simulink model "Series_connected_PV_modules"  (Simulink 8.4)
settings: Solver=FixedStepDiscrete  StartTime=0.0  StopTime=1  FixedStep=1e-4  RelTol=1e-3
libraries: simulink x1
(part 1 of 2)
settings Model: Creator=amaki  LastModifiedBy=lappalak
settings DebuggingCC: AlgebraicLoopMsg=none  StrictBusMsg=Warning
settings ConfigurationSet: Description=SimMechanics 2G

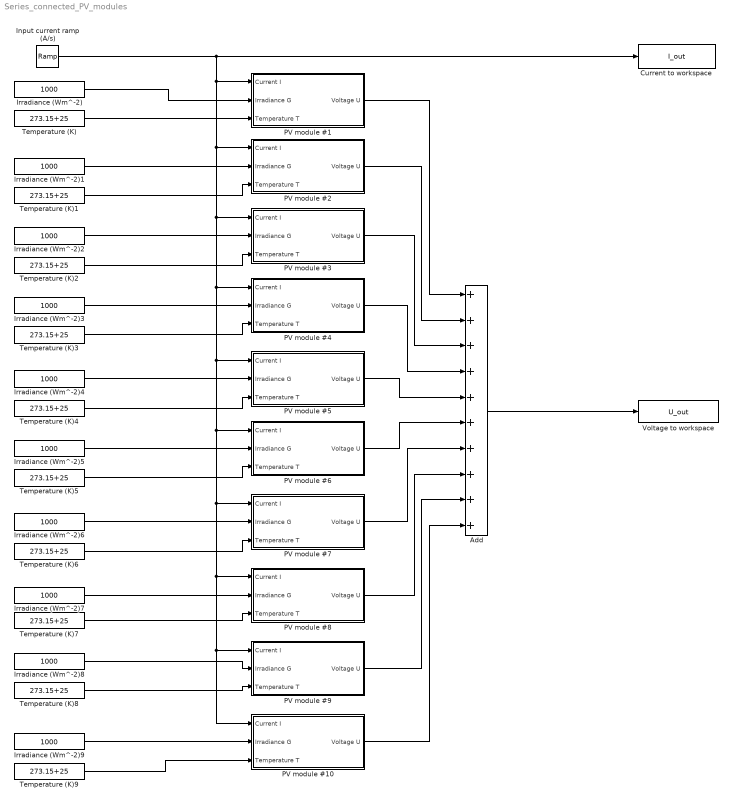
== system Series_connected_PV_modules ==
  Add : Sum  Inputs=++++++++++
  Current to workspace : ToWorkspace  VariableName=I_out  SampleTime=-1
  Input current ramp (A/s) : simulink/Sources/Ramp  slope=10  start=0  X0=0
  Irradiance (Wm^-2){,1..9} (10 alike) : Constant  Value=1000
  PV module #1 : Subsystem  mask{Isc_stc=8.02, Uoc_stc=33.1, G_stc=1000, T_stc=273.15+25, Ns=54, Rs=0.33, Rsh=188, A=1.3, Ku=-0.1242, Ki=0.0047, k=1.3806503e-23, q=1.60217646e-19}
      mask prompts: Isc_stc "STC short-circuit current"; Uoc_stc "STC open-circuit voltage"; G_stc "STC irradiance"; T_stc "STC temperature"; Ns "Number of cells"; Rs "Series resistance Rs"; Rsh "Shunt resistance Rsh"; A "Ideality factor A"; Ku "Temp. coeff. of OC Ku"; Ki "Temp. coeff. of SC Ki"; k "Boltzmann constant"; q "Elementary charge"
  PV module #10 : Subsystem  mask{Isc_stc=8.02, Uoc_stc=33.1, G_stc=1000, T_stc=273.15+25, Ns=54, Rs=0.33, Rsh=188, A=1.3, Ku=-0.1242, Ki=0.0047, k=1.3806503e-23, q=1.60217646e-19}
      mask prompts: Isc_stc "STC short-circuit current"; Uoc_stc "STC open-circuit voltage"; G_stc "STC irradiance"; T_stc "STC temperature"; Ns "Number of cells"; Rs "Series resistance Rs"; Rsh "Shunt resistance Rsh"; A "Ideality factor A"; Ku "Temp. coeff. of OC Ku"; Ki "Temp. coeff. of SC Ki"; k "Boltzmann constant"; q "Elementary charge"
  PV module #2 : Subsystem  mask{Isc_stc=8.02, Uoc_stc=33.1, G_stc=1000, T_stc=273.15+25, Ns=54, Rs=0.33, Rsh=188, A=1.3, Ku=-0.1242, Ki=0.0047, k=1.3806503e-23, q=1.60217646e-19}
      mask prompts: Isc_stc "STC short-circuit current"; Uoc_stc "STC open-circuit voltage"; G_stc "STC irradiance"; T_stc "STC temperature"; Ns "Number of cells"; Rs "Series resistance Rs"; Rsh "Shunt resistance Rsh"; A "Ideality factor A"; Ku "Temp. coeff. of OC Ku"; Ki "Temp. coeff. of SC Ki"; k "Boltzmann constant"; q "Elementary charge"
  PV module #3 : Subsystem  mask{Isc_stc=8.02, Uoc_stc=33.1, G_stc=1000, T_stc=273.15+25, Ns=54, Rs=0.33, Rsh=188, A=1.3, Ku=-0.1242, Ki=0.0047, k=1.3806503e-23, q=1.60217646e-19}
      mask prompts: Isc_stc "STC short-circuit current"; Uoc_stc "STC open-circuit voltage"; G_stc "STC irradiance"; T_stc "STC temperature"; Ns "Number of cells"; Rs "Series resistance Rs"; Rsh "Shunt resistance Rsh"; A "Ideality factor A"; Ku "Temp. coeff. of OC Ku"; Ki "Temp. coeff. of SC Ki"; k "Boltzmann constant"; q "Elementary charge"
  PV module #4 : Subsystem  mask{Isc_stc=8.02, Uoc_stc=33.1, G_stc=1000, T_stc=273.15+25, Ns=54, Rs=0.33, Rsh=188, A=1.3, Ku=-0.1242, Ki=0.0047, k=1.3806503e-23, q=1.60217646e-19}
      mask prompts: Isc_stc "STC short-circuit current"; Uoc_stc "STC open-circuit voltage"; G_stc "STC irradiance"; T_stc "STC temperature"; Ns "Number of cells"; Rs "Series resistance Rs"; Rsh "Shunt resistance Rsh"; A "Ideality factor A"; Ku "Temp. coeff. of OC Ku"; Ki "Temp. coeff. of SC Ki"; k "Boltzmann constant"; q "Elementary charge"
  PV module #5 : Subsystem  mask{Isc_stc=8.02, Uoc_stc=33.1, G_stc=1000, T_stc=273.15+25, Ns=54, Rs=0.33, Rsh=188, A=1.3, Ku=-0.1242, Ki=0.0047, k=1.3806503e-23, q=1.60217646e-19}
      mask prompts: Isc_stc "STC short-circuit current"; Uoc_stc "STC open-circuit voltage"; G_stc "STC irradiance"; T_stc "STC temperature"; Ns "Number of cells"; Rs "Series resistance Rs"; Rsh "Shunt resistance Rsh"; A "Ideality factor A"; Ku "Temp. coeff. of OC Ku"; Ki "Temp. coeff. of SC Ki"; k "Boltzmann constant"; q "Elementary charge"
  PV module #6 : Subsystem  mask{Isc_stc=8.02, Uoc_stc=33.1, G_stc=1000, T_stc=273.15+25, Ns=54, Rs=0.33, Rsh=188, A=1.3, Ku=-0.1242, Ki=0.0047, k=1.3806503e-23, q=1.60217646e-19}
      mask prompts: Isc_stc "STC short-circuit current"; Uoc_stc "STC open-circuit voltage"; G_stc "STC irradiance"; T_stc "STC temperature"; Ns "Number of cells"; Rs "Series resistance Rs"; Rsh "Shunt resistance Rsh"; A "Ideality factor A"; Ku "Temp. coeff. of OC Ku"; Ki "Temp. coeff. of SC Ki"; k "Boltzmann constant"; q "Elementary charge"
  PV module #7 : Subsystem  mask{Isc_stc=8.02, Uoc_stc=33.1, G_stc=1000, T_stc=273.15+25, Ns=54, Rs=0.33, Rsh=188, A=1.3, Ku=-0.1242, Ki=0.0047, k=1.3806503e-23, q=1.60217646e-19}
      mask prompts: Isc_stc "STC short-circuit current"; Uoc_stc "STC open-circuit voltage"; G_stc "STC irradiance"; T_stc "STC temperature"; Ns "Number of cells"; Rs "Series resistance Rs"; Rsh "Shunt resistance Rsh"; A "Ideality factor A"; Ku "Temp. coeff. of OC Ku"; Ki "Temp. coeff. of SC Ki"; k "Boltzmann constant"; q "Elementary charge"
  PV module #8 : Subsystem  mask{Isc_stc=8.02, Uoc_stc=33.1, G_stc=1000, T_stc=273.15+25, Ns=54, Rs=0.33, Rsh=188, A=1.3, Ku=-0.1242, Ki=0.0047, k=1.3806503e-23, q=1.60217646e-19}
      mask prompts: Isc_stc "STC short-circuit current"; Uoc_stc "STC open-circuit voltage"; G_stc "STC irradiance"; T_stc "STC temperature"; Ns "Number of cells"; Rs "Series resistance Rs"; Rsh "Shunt resistance Rsh"; A "Ideality factor A"; Ku "Temp. coeff. of OC Ku"; Ki "Temp. coeff. of SC Ki"; k "Boltzmann constant"; q "Elementary charge"
  PV module #9 : Subsystem  mask{Isc_stc=8.02, Uoc_stc=33.1, G_stc=1000, T_stc=273.15+25, Ns=54, Rs=0.33, Rsh=188, A=1.3, Ku=-0.1242, Ki=0.0047, k=1.3806503e-23, q=1.60217646e-19}
      mask prompts: Isc_stc "STC short-circuit current"; Uoc_stc "STC open-circuit voltage"; G_stc "STC irradiance"; T_stc "STC temperature"; Ns "Number of cells"; Rs "Series resistance Rs"; Rsh "Shunt resistance Rsh"; A "Ideality factor A"; Ku "Temp. coeff. of OC Ku"; Ki "Temp. coeff. of SC Ki"; k "Boltzmann constant"; q "Elementary charge"
  Temperature (K){,1..9} (10 alike) : Constant  Value=273.15+25
  Voltage to workspace : ToWorkspace  VariableName=U_out  SampleTime=-1
  wires:
  Temperature (K)/1 -> PV module #1/3(Temperature T)
  Input current ramp (A/s)/1 -> Current to workspace/1, PV module #1/1(Current I), PV module #2/1(Current I), PV module #3/1(Current I), PV module #4/1(Current I), PV module #5/1(Current I), PV module #6/1(Current I), PV module #7/1(Current I), PV module #8/1(Current I), PV module #9/1(Current I), PV module #10/1(Current I)
  Irradiance (Wm^-2)/1 -> PV module #1/2(Irradiance G)
  Irradiance (Wm^-2)1/1 -> PV module #2/2(Irradiance G)
  Irradiance (Wm^-2)2/1 -> PV module #3/2(Irradiance G)
  Irradiance (Wm^-2)3/1 -> PV module #4/2(Irradiance G)
  Irradiance (Wm^-2)4/1 -> PV module #5/2(Irradiance G)
  Irradiance (Wm^-2)5/1 -> PV module #6/2(Irradiance G)
  Irradiance (Wm^-2)6/1 -> PV module #7/2(Irradiance G)
  Irradiance (Wm^-2)7/1 -> PV module #8/2(Irradiance G)
  Irradiance (Wm^-2)9/1 -> PV module #10/2(Irradiance G)
  Temperature (K)1/1 -> PV module #2/3(Temperature T)
  Temperature (K)2/1 -> PV module #3/3(Temperature T)
  Temperature (K)3/1 -> PV module #4/3(Temperature T)
  Temperature (K)4/1 -> PV module #5/3(Temperature T)
  Temperature (K)5/1 -> PV module #6/3(Temperature T)
  Temperature (K)7/1 -> PV module #8/3(Temperature T)
  Temperature (K)9/1 -> PV module #10/3(Temperature T)
  Temperature (K)6/1 -> PV module #7/3(Temperature T)
  PV module #1/1(Voltage U) -> Add/1
  PV module #2/1(Voltage U) -> Add/2
  PV module #3/1(Voltage U) -> Add/3
  PV module #4/1(Voltage U) -> Add/4
  PV module #5/1(Voltage U) -> Add/5
  PV module #6/1(Voltage U) -> Add/6
  PV module #7/1(Voltage U) -> Add/7
  PV module #8/1(Voltage U) -> Add/8
  PV module #9/1(Voltage U) -> Add/9
  PV module #10/1(Voltage U) -> Add/10
  Add/1 -> Voltage to workspace/1
  Irradiance (Wm^-2)8/1 -> PV module #9/2(Irradiance G)
  Temperature (K)8/1 -> PV module #9/3(Temperature T)

== system Series_connected_PV_modules/PV module #1 ==
  Current I : Inport
  Irradiance G : Inport  Port=2
  Temperature T : Inport  Port=3
  Add1 : Sum  Inputs=-+
  Bypass diode : Subsystem  mask{k=1.3806503e-23, q=1.60217646e-19, Rs_bypass=0.02}
      mask prompts: k "Boltzmann constant"; q "Elementary charge"; Rs_bypass "Series resistance"
  MinMax : MinMax  Function=max  Inputs=2
  Pv module : Subsystem
  Voltage U : Outport
  wires:
  MinMax/1 -> Voltage U/1
  Add1/1 -> Bypass diode/1(I)
  Bypass diode/1(Ubypass) -> MinMax/2
  Pv module/2(Isc) -> Add1/1
  Pv module/1(U) -> MinMax/1
  Irradiance G/1 -> Pv module/1(G)
  Temperature T/1 -> Pv module/2(T)
  Current I/1 -> Pv module/3(I), Add1/2

== system Series_connected_PV_modules/PV module #10 ==
  Current I : Inport
  Irradiance G : Inport  Port=2
  Temperature T : Inport  Port=3
  Add1 : Sum  Inputs=-+
  Bypass diode : Subsystem  mask{k=1.3806503e-23, q=1.60217646e-19, Rs_bypass=0.02}
      mask prompts: k "Boltzmann constant"; q "Elementary charge"; Rs_bypass "Series resistance"
  MinMax : MinMax  Function=max  Inputs=2
  Pv module : Subsystem
  Voltage U : Outport
  wires:
  MinMax/1 -> Voltage U/1
  Add1/1 -> Bypass diode/1(I)
  Bypass diode/1(Ubypass) -> MinMax/2
  Pv module/2(Isc) -> Add1/1
  Pv module/1(U) -> MinMax/1
  Irradiance G/1 -> Pv module/1(G)
  Temperature T/1 -> Pv module/2(T)
  Current I/1 -> Pv module/3(I), Add1/2

== system Series_connected_PV_modules/PV module #2 ==
  Current I : Inport
  Irradiance G : Inport  Port=2
  Temperature T : Inport  Port=3
  Add1 : Sum  Inputs=-+
  Bypass diode : Subsystem  mask{k=1.3806503e-23, q=1.60217646e-19, Rs_bypass=0.02}
      mask prompts: k "Boltzmann constant"; q "Elementary charge"; Rs_bypass "Series resistance"
  MinMax : MinMax  Function=max  Inputs=2
  Pv module : Subsystem
  Voltage U : Outport
  wires:
  Current I/1 -> Add1/2, Pv module/3(I)
  Temperature T/1 -> Pv module/2(T)
  Irradiance G/1 -> Pv module/1(G)
  Pv module/1(U) -> MinMax/1
  Pv module/2(Isc) -> Add1/1
  Bypass diode/1(Ubypass) -> MinMax/2
  Add1/1 -> Bypass diode/1(I)
  MinMax/1 -> Voltage U/1

== system Series_connected_PV_modules/PV module #3 ==
  Current I : Inport
  Irradiance G : Inport  Port=2
  Temperature T : Inport  Port=3
  Add1 : Sum  Inputs=-+
  Bypass diode : Subsystem  mask{k=1.3806503e-23, q=1.60217646e-19, Rs_bypass=0.02}
      mask prompts: k "Boltzmann constant"; q "Elementary charge"; Rs_bypass "Series resistance"
  MinMax : MinMax  Function=max  Inputs=2
  Pv module : Subsystem
  Voltage U : Outport
  wires:
  MinMax/1 -> Voltage U/1
  Add1/1 -> Bypass diode/1(I)
  Bypass diode/1(Ubypass) -> MinMax/2
  Pv module/2(Isc) -> Add1/1
  Pv module/1(U) -> MinMax/1
  Irradiance G/1 -> Pv module/1(G)
  Temperature T/1 -> Pv module/2(T)
  Current I/1 -> Pv module/3(I), Add1/2

== system Series_connected_PV_modules/PV module #4 ==
  Current I : Inport
  Irradiance G : Inport  Port=2
  Temperature T : Inport  Port=3
  Add1 : Sum  Inputs=-+
  Bypass diode : Subsystem  mask{k=1.3806503e-23, q=1.60217646e-19, Rs_bypass=0.02}
      mask prompts: k "Boltzmann constant"; q "Elementary charge"; Rs_bypass "Series resistance"
  MinMax : MinMax  Function=max  Inputs=2
  Pv module : Subsystem
  Voltage U : Outport
  wires:
  Current I/1 -> Add1/2, Pv module/3(I)
  Temperature T/1 -> Pv module/2(T)
  Irradiance G/1 -> Pv module/1(G)
  Pv module/1(U) -> MinMax/1
  Pv module/2(Isc) -> Add1/1
  Bypass diode/1(Ubypass) -> MinMax/2
  Add1/1 -> Bypass diode/1(I)
  MinMax/1 -> Voltage U/1

== system Series_connected_PV_modules/PV module #5 ==
  Current I : Inport
  Irradiance G : Inport  Port=2
  Temperature T : Inport  Port=3
  Add1 : Sum  Inputs=-+
  Bypass diode : Subsystem  mask{k=1.3806503e-23, q=1.60217646e-19, Rs_bypass=0.02}
      mask prompts: k "Boltzmann constant"; q "Elementary charge"; Rs_bypass "Series resistance"
  MinMax : MinMax  Function=max  Inputs=2
  Pv module : Subsystem
  Voltage U : Outport
  wires:
  MinMax/1 -> Voltage U/1
  Add1/1 -> Bypass diode/1(I)
  Bypass diode/1(Ubypass) -> MinMax/2
  Pv module/2(Isc) -> Add1/1
  Pv module/1(U) -> MinMax/1
  Irradiance G/1 -> Pv module/1(G)
  Temperature T/1 -> Pv module/2(T)
  Current I/1 -> Pv module/3(I), Add1/2

== system Series_connected_PV_modules/PV module #6 ==
  Current I : Inport
  Irradiance G : Inport  Port=2
  Temperature T : Inport  Port=3
  Add1 : Sum  Inputs=-+
  Bypass diode : Subsystem  mask{k=1.3806503e-23, q=1.60217646e-19, Rs_bypass=0.02}
      mask prompts: k "Boltzmann constant"; q "Elementary charge"; Rs_bypass "Series resistance"
  MinMax : MinMax  Function=max  Inputs=2
  Pv module : Subsystem
  Voltage U : Outport
  wires:
  Current I/1 -> Add1/2, Pv module/3(I)
  Temperature T/1 -> Pv module/2(T)
  Irradiance G/1 -> Pv module/1(G)
  Pv module/1(U) -> MinMax/1
  Pv module/2(Isc) -> Add1/1
  Bypass diode/1(Ubypass) -> MinMax/2
  Add1/1 -> Bypass diode/1(I)
  MinMax/1 -> Voltage U/1

== system Series_connected_PV_modules/PV module #7 ==
  Current I : Inport
  Irradiance G : Inport  Port=2
  Temperature T : Inport  Port=3
  Add1 : Sum  Inputs=-+
  Bypass diode : Subsystem  mask{k=1.3806503e-23, q=1.60217646e-19, Rs_bypass=0.02}
      mask prompts: k "Boltzmann constant"; q "Elementary charge"; Rs_bypass "Series resistance"
  MinMax : MinMax  Function=max  Inputs=2
  Pv module : Subsystem
  Voltage U : Outport
  wires:
  Current I/1 -> Add1/2, Pv module/3(I)
  Temperature T/1 -> Pv module/2(T)
  Irradiance G/1 -> Pv module/1(G)
  Pv module/1(U) -> MinMax/1
  Pv module/2(Isc) -> Add1/1
  Bypass diode/1(Ubypass) -> MinMax/2
  Add1/1 -> Bypass diode/1(I)
  MinMax/1 -> Voltage U/1

== system Series_connected_PV_modules/PV module #8 ==
  Current I : Inport
  Irradiance G : Inport  Port=2
  Temperature T : Inport  Port=3
  Add1 : Sum  Inputs=-+
  Bypass diode : Subsystem  mask{k=1.3806503e-23, q=1.60217646e-19, Rs_bypass=0.02}
      mask prompts: k "Boltzmann constant"; q "Elementary charge"; Rs_bypass "Series resistance"
  MinMax : MinMax  Function=max  Inputs=2
  Pv module : Subsystem
  Voltage U : Outport
  wires:
  MinMax/1 -> Voltage U/1
  Add1/1 -> Bypass diode/1(I)
  Bypass diode/1(Ubypass) -> MinMax/2
  Pv module/2(Isc) -> Add1/1
  Pv module/1(U) -> MinMax/1
  Irradiance G/1 -> Pv module/1(G)
  Temperature T/1 -> Pv module/2(T)
  Current I/1 -> Pv module/3(I), Add1/2

== system Series_connected_PV_modules/PV module #9 ==
  Current I : Inport
  Irradiance G : Inport  Port=2
  Temperature T : Inport  Port=3
  Add1 : Sum  Inputs=-+
  Bypass diode : Subsystem  mask{k=1.3806503e-23, q=1.60217646e-19, Rs_bypass=0.02}
      mask prompts: k "Boltzmann constant"; q "Elementary charge"; Rs_bypass "Series resistance"
  MinMax : MinMax  Function=max  Inputs=2
  Pv module : Subsystem
  Voltage U : Outport
  wires:
  Current I/1 -> Add1/2, Pv module/3(I)
  Temperature T/1 -> Pv module/2(T)
  Irradiance G/1 -> Pv module/1(G)
  Pv module/1(U) -> MinMax/1
  Pv module/2(Isc) -> Add1/1
  Bypass diode/1(Ubypass) -> MinMax/2
  Add1/1 -> Bypass diode/1(I)
  MinMax/1 -> Voltage U/1

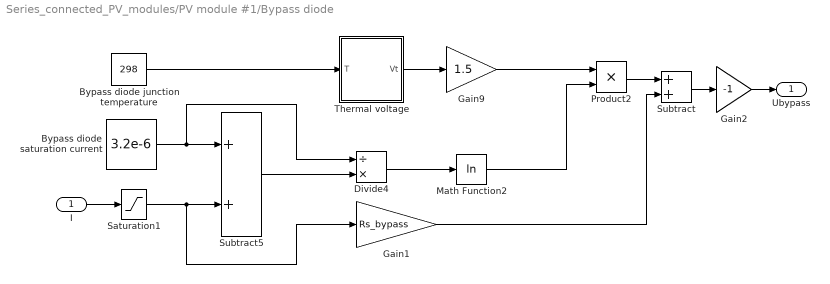
== system Series_connected_PV_modules/PV module #1/Bypass diode ==
  I : Inport
  Bypass diode junction temperature : Constant  Value=298
  Bypass diode saturation current : Constant  Value=3.2e-6
  Divide4 : Product  Inputs=/*
  Gain1 : Gain  Gain=Rs_bypass
  Gain2 : Gain  Gain=-1
  Gain9 : Gain  Gain=1.5
  Math Function2 : Math  Operator=log  SaturateOnIntegerOverflow=on
  Product2 : Product  RndMeth=Zero
  Saturation1 : Saturate  UpperLimit=1e24  LowerLimit=0
  Subtract : Sum
  Subtract5 : Sum
  Thermal voltage : Subsystem
  Ubypass : Outport
  wires:
  Gain2/1 -> Ubypass/1
  Subtract/1 -> Gain2/1
  Saturation1/1 -> Gain1/1, Subtract5/2
  Subtract5/1 -> Divide4/2
  Divide4/1 -> Math Function2/1
  Bypass diode junction temperature/1 -> Thermal voltage/1(T)
  Gain1/1 -> Subtract/2
  Product2/1 -> Subtract/1
  I/1 -> Saturation1/1
  Bypass diode saturation current/1 -> Divide4/1, Subtract5/1
  Thermal voltage/1(Vt) -> Gain9/1
  Gain9/1 -> Product2/1
  Math Function2/1 -> Product2/2

== system Series_connected_PV_modules/PV module #1/Pv module ==
  G : Inport
  T : Inport  Port=2
  I : Inport  Port=3
  Add1 : Sum  Inputs=+--
  Gain1 : Gain  Gain=Rsh
  Gain3 : Gain  Gain=(Rsh+Rs)/Rsh
  Subsystem : Subsystem
  Subsystem1 : Subsystem
  U : Outport
  Isc : Outport  Port=2
  wires:
  Subsystem/1(Isc) -> Isc/1
  Gain1/1 -> U/1, Subsystem1/2(U)
  Add1/1 -> Gain1/1
  Gain3/1 -> Add1/3
  I/1 -> Gain3/1, Subsystem1/3(I)
  Subsystem1/1(Id) -> Add1/2
  T/1 -> Subsystem1/1(T), Subsystem/2(T)
  G/1 -> Subsystem/1(G)
  Subsystem/2(Ipv) -> Add1/1

== system Series_connected_PV_modules/PV module #10/Bypass diode ==
  I : Inport
  Bypass diode junction temperature : Constant  Value=298
  Bypass diode saturation current : Constant  Value=3.2e-6
  Divide4 : Product  Inputs=/*
  Gain1 : Gain  Gain=Rs_bypass
  Gain2 : Gain  Gain=-1
  Gain9 : Gain  Gain=1.5
  Math Function2 : Math  Operator=log  SaturateOnIntegerOverflow=on
  Product2 : Product  RndMeth=Zero
  Saturation1 : Saturate  UpperLimit=1e24  LowerLimit=0
  Subtract : Sum
  Subtract5 : Sum
  Thermal voltage : Subsystem
  Ubypass : Outport
  wires:
  Gain2/1 -> Ubypass/1
  Subtract/1 -> Gain2/1
  Saturation1/1 -> Gain1/1, Subtract5/2
  Subtract5/1 -> Divide4/2
  Divide4/1 -> Math Function2/1
  Bypass diode junction temperature/1 -> Thermal voltage/1(T)
  Gain1/1 -> Subtract/2
  Product2/1 -> Subtract/1
  I/1 -> Saturation1/1
  Bypass diode saturation current/1 -> Divide4/1, Subtract5/1
  Thermal voltage/1(Vt) -> Gain9/1
  Gain9/1 -> Product2/1
  Math Function2/1 -> Product2/2

== system Series_connected_PV_modules/PV module #10/Pv module ==
  G : Inport
  T : Inport  Port=2
  I : Inport  Port=3
  Add1 : Sum  Inputs=+--
  Gain1 : Gain  Gain=Rsh
  Gain3 : Gain  Gain=(Rsh+Rs)/Rsh
  Subsystem : Subsystem
  Subsystem1 : Subsystem
  U : Outport
  Isc : Outport  Port=2
  wires:
  Subsystem/1(Isc) -> Isc/1
  Gain1/1 -> U/1, Subsystem1/2(U)
  Add1/1 -> Gain1/1
  Gain3/1 -> Add1/3
  I/1 -> Gain3/1, Subsystem1/3(I)
  Subsystem1/1(Id) -> Add1/2
  T/1 -> Subsystem1/1(T), Subsystem/2(T)
  G/1 -> Subsystem/1(G)
  Subsystem/2(Ipv) -> Add1/1

== system Series_connected_PV_modules/PV module #2/Bypass diode ==
  I : Inport
  Bypass diode junction temperature : Constant  Value=298
  Bypass diode saturation current : Constant  Value=3.2e-6
  Divide4 : Product  Inputs=/*
  Gain1 : Gain  Gain=Rs_bypass
  Gain2 : Gain  Gain=-1
  Gain9 : Gain  Gain=1.5
  Math Function2 : Math  Operator=log  SaturateOnIntegerOverflow=on
  Product2 : Product  RndMeth=Zero
  Saturation1 : Saturate  UpperLimit=1e24  LowerLimit=0
  Subtract : Sum
  Subtract5 : Sum
  Thermal voltage : Subsystem
  Ubypass : Outport
  wires:
  Math Function2/1 -> Product2/2
  Gain9/1 -> Product2/1
  Thermal voltage/1(Vt) -> Gain9/1
  Bypass diode saturation current/1 -> Subtract5/1, Divide4/1
  I/1 -> Saturation1/1
  Product2/1 -> Subtract/1
  Gain1/1 -> Subtract/2
  Bypass diode junction temperature/1 -> Thermal voltage/1(T)
  Divide4/1 -> Math Function2/1
  Subtract5/1 -> Divide4/2
  Saturation1/1 -> Subtract5/2, Gain1/1
  Subtract/1 -> Gain2/1
  Gain2/1 -> Ubypass/1

== system Series_connected_PV_modules/PV module #2/Pv module ==
  G : Inport
  T : Inport  Port=2
  I : Inport  Port=3
  Add1 : Sum  Inputs=+--
  Gain1 : Gain  Gain=Rsh
  Gain3 : Gain  Gain=(Rsh+Rs)/Rsh
  Subsystem : Subsystem
  Subsystem1 : Subsystem
  U : Outport
  Isc : Outport  Port=2
  wires:
  Subsystem/2(Ipv) -> Add1/1
  G/1 -> Subsystem/1(G)
  T/1 -> Subsystem/2(T), Subsystem1/1(T)
  Subsystem1/1(Id) -> Add1/2
  I/1 -> Subsystem1/3(I), Gain3/1
  Gain3/1 -> Add1/3
  Add1/1 -> Gain1/1
  Gain1/1 -> Subsystem1/2(U), U/1
  Subsystem/1(Isc) -> Isc/1

== system Series_connected_PV_modules/PV module #3/Bypass diode ==
  I : Inport
  Bypass diode junction temperature : Constant  Value=298
  Bypass diode saturation current : Constant  Value=3.2e-6
  Divide4 : Product  Inputs=/*
  Gain1 : Gain  Gain=Rs_bypass
  Gain2 : Gain  Gain=-1
  Gain9 : Gain  Gain=1.5
  Math Function2 : Math  Operator=log  SaturateOnIntegerOverflow=on
  Product2 : Product  RndMeth=Zero
  Saturation1 : Saturate  UpperLimit=1e24  LowerLimit=0
  Subtract : Sum
  Subtract5 : Sum
  Thermal voltage : Subsystem
  Ubypass : Outport
  wires:
  Gain2/1 -> Ubypass/1
  Subtract/1 -> Gain2/1
  Saturation1/1 -> Gain1/1, Subtract5/2
  Subtract5/1 -> Divide4/2
  Divide4/1 -> Math Function2/1
  Bypass diode junction temperature/1 -> Thermal voltage/1(T)
  Gain1/1 -> Subtract/2
  Product2/1 -> Subtract/1
  I/1 -> Saturation1/1
  Bypass diode saturation current/1 -> Divide4/1, Subtract5/1
  Thermal voltage/1(Vt) -> Gain9/1
  Gain9/1 -> Product2/1
  Math Function2/1 -> Product2/2

== system Series_connected_PV_modules/PV module #3/Pv module ==
  G : Inport
  T : Inport  Port=2
  I : Inport  Port=3
  Add1 : Sum  Inputs=+--
  Gain1 : Gain  Gain=Rsh
  Gain3 : Gain  Gain=(Rsh+Rs)/Rsh
  Subsystem : Subsystem
  Subsystem1 : Subsystem
  U : Outport
  Isc : Outport  Port=2
  wires:
  Subsystem/1(Isc) -> Isc/1
  Gain1/1 -> U/1, Subsystem1/2(U)
  Add1/1 -> Gain1/1
  Gain3/1 -> Add1/3
  I/1 -> Gain3/1, Subsystem1/3(I)
  Subsystem1/1(Id) -> Add1/2
  T/1 -> Subsystem1/1(T), Subsystem/2(T)
  G/1 -> Subsystem/1(G)
  Subsystem/2(Ipv) -> Add1/1

== system Series_connected_PV_modules/PV module #4/Bypass diode ==
  I : Inport
  Bypass diode junction temperature : Constant  Value=298
  Bypass diode saturation current : Constant  Value=3.2e-6
  Divide4 : Product  Inputs=/*
  Gain1 : Gain  Gain=Rs_bypass
  Gain2 : Gain  Gain=-1
  Gain9 : Gain  Gain=1.5
  Math Function2 : Math  Operator=log  SaturateOnIntegerOverflow=on
  Product2 : Product  RndMeth=Zero
  Saturation1 : Saturate  UpperLimit=1e24  LowerLimit=0
  Subtract : Sum
  Subtract5 : Sum
  Thermal voltage : Subsystem
  Ubypass : Outport
  wires:
  Math Function2/1 -> Product2/2
  Gain9/1 -> Product2/1
  Thermal voltage/1(Vt) -> Gain9/1
  Bypass diode saturation current/1 -> Subtract5/1, Divide4/1
  I/1 -> Saturation1/1
  Product2/1 -> Subtract/1
  Gain1/1 -> Subtract/2
  Bypass diode junction temperature/1 -> Thermal voltage/1(T)
  Divide4/1 -> Math Function2/1
  Subtract5/1 -> Divide4/2
  Saturation1/1 -> Subtract5/2, Gain1/1
  Subtract/1 -> Gain2/1
  Gain2/1 -> Ubypass/1

== system Series_connected_PV_modules/PV module #4/Pv module ==
  G : Inport
  T : Inport  Port=2
  I : Inport  Port=3
  Add1 : Sum  Inputs=+--
  Gain1 : Gain  Gain=Rsh
  Gain3 : Gain  Gain=(Rsh+Rs)/Rsh
  Subsystem : Subsystem
  Subsystem1 : Subsystem
  U : Outport
  Isc : Outport  Port=2
  wires:
  Subsystem/2(Ipv) -> Add1/1
  G/1 -> Subsystem/1(G)
  T/1 -> Subsystem/2(T), Subsystem1/1(T)
  Subsystem1/1(Id) -> Add1/2
  I/1 -> Subsystem1/3(I), Gain3/1
  Gain3/1 -> Add1/3
  Add1/1 -> Gain1/1
  Gain1/1 -> Subsystem1/2(U), U/1
  Subsystem/1(Isc) -> Isc/1

== system Series_connected_PV_modules/PV module #5/Bypass diode ==
  I : Inport
  Bypass diode junction temperature : Constant  Value=298
  Bypass diode saturation current : Constant  Value=3.2e-6
  Divide4 : Product  Inputs=/*
  Gain1 : Gain  Gain=Rs_bypass
  Gain2 : Gain  Gain=-1
  Gain9 : Gain  Gain=1.5
  Math Function2 : Math  Operator=log  SaturateOnIntegerOverflow=on
  Product2 : Product  RndMeth=Zero
  Saturation1 : Saturate  UpperLimit=1e24  LowerLimit=0
  Subtract : Sum
  Subtract5 : Sum
  Thermal voltage : Subsystem
  Ubypass : Outport
  wires:
  Gain2/1 -> Ubypass/1
  Subtract/1 -> Gain2/1
  Saturation1/1 -> Gain1/1, Subtract5/2
  Subtract5/1 -> Divide4/2
  Divide4/1 -> Math Function2/1
  Bypass diode junction temperature/1 -> Thermal voltage/1(T)
  Gain1/1 -> Subtract/2
  Product2/1 -> Subtract/1
  I/1 -> Saturation1/1
  Bypass diode saturation current/1 -> Divide4/1, Subtract5/1
  Thermal voltage/1(Vt) -> Gain9/1
  Gain9/1 -> Product2/1
  Math Function2/1 -> Product2/2

== system Series_connected_PV_modules/PV module #5/Pv module ==
  G : Inport
  T : Inport  Port=2
  I : Inport  Port=3
  Add1 : Sum  Inputs=+--
  Gain1 : Gain  Gain=Rsh
  Gain3 : Gain  Gain=(Rsh+Rs)/Rsh
  Subsystem : Subsystem
  Subsystem1 : Subsystem
  U : Outport
  Isc : Outport  Port=2
  wires:
  Subsystem/1(Isc) -> Isc/1
  Gain1/1 -> U/1, Subsystem1/2(U)
  Add1/1 -> Gain1/1
  Gain3/1 -> Add1/3
  I/1 -> Gain3/1, Subsystem1/3(I)
  Subsystem1/1(Id) -> Add1/2
  T/1 -> Subsystem1/1(T), Subsystem/2(T)
  G/1 -> Subsystem/1(G)
  Subsystem/2(Ipv) -> Add1/1

== system Series_connected_PV_modules/PV module #6/Bypass diode ==
  I : Inport
  Bypass diode junction temperature : Constant  Value=298
  Bypass diode saturation current : Constant  Value=3.2e-6
  Divide4 : Product  Inputs=/*
  Gain1 : Gain  Gain=Rs_bypass
  Gain2 : Gain  Gain=-1
  Gain9 : Gain  Gain=1.5
  Math Function2 : Math  Operator=log  SaturateOnIntegerOverflow=on
  Product2 : Product  RndMeth=Zero
  Saturation1 : Saturate  UpperLimit=1e24  LowerLimit=0
  Subtract : Sum
  Subtract5 : Sum
  Thermal voltage : Subsystem
  Ubypass : Outport
  wires:
  Math Function2/1 -> Product2/2
  Gain9/1 -> Product2/1
  Thermal voltage/1(Vt) -> Gain9/1
  Bypass diode saturation current/1 -> Subtract5/1, Divide4/1
  I/1 -> Saturation1/1
  Product2/1 -> Subtract/1
  Gain1/1 -> Subtract/2
  Bypass diode junction temperature/1 -> Thermal voltage/1(T)
  Divide4/1 -> Math Function2/1
  Subtract5/1 -> Divide4/2
  Saturation1/1 -> Subtract5/2, Gain1/1
  Subtract/1 -> Gain2/1
  Gain2/1 -> Ubypass/1

== system Series_connected_PV_modules/PV module #6/Pv module ==
  G : Inport
  T : Inport  Port=2
  I : Inport  Port=3
  Add1 : Sum  Inputs=+--
  Gain1 : Gain  Gain=Rsh
  Gain3 : Gain  Gain=(Rsh+Rs)/Rsh
  Subsystem : Subsystem
  Subsystem1 : Subsystem
  U : Outport
  Isc : Outport  Port=2
  wires:
  Subsystem/2(Ipv) -> Add1/1
  G/1 -> Subsystem/1(G)
  T/1 -> Subsystem/2(T), Subsystem1/1(T)
  Subsystem1/1(Id) -> Add1/2
  I/1 -> Subsystem1/3(I), Gain3/1
  Gain3/1 -> Add1/3
  Add1/1 -> Gain1/1
  Gain1/1 -> Subsystem1/2(U), U/1
  Subsystem/1(Isc) -> Isc/1

== system Series_connected_PV_modules/PV module #7/Bypass diode ==
  I : Inport
  Bypass diode junction temperature : Constant  Value=298
  Bypass diode saturation current : Constant  Value=3.2e-6
  Divide4 : Product  Inputs=/*
  Gain1 : Gain  Gain=Rs_bypass
  Gain2 : Gain  Gain=-1
  Gain9 : Gain  Gain=1.5
  Math Function2 : Math  Operator=log  SaturateOnIntegerOverflow=on
  Product2 : Product  RndMeth=Zero
  Saturation1 : Saturate  UpperLimit=1e24  LowerLimit=0
  Subtract : Sum
  Subtract5 : Sum
  Thermal voltage : Subsystem
  Ubypass : Outport
  wires:
  Math Function2/1 -> Product2/2
  Gain9/1 -> Product2/1
  Thermal voltage/1(Vt) -> Gain9/1
  Bypass diode saturation current/1 -> Subtract5/1, Divide4/1
  I/1 -> Saturation1/1
  Product2/1 -> Subtract/1
  Gain1/1 -> Subtract/2
  Bypass diode junction temperature/1 -> Thermal voltage/1(T)
  Divide4/1 -> Math Function2/1
  Subtract5/1 -> Divide4/2
  Saturation1/1 -> Subtract5/2, Gain1/1
  Subtract/1 -> Gain2/1
  Gain2/1 -> Ubypass/1

== system Series_connected_PV_modules/PV module #7/Pv module ==
  G : Inport
  T : Inport  Port=2
  I : Inport  Port=3
  Add1 : Sum  Inputs=+--
  Gain1 : Gain  Gain=Rsh
  Gain3 : Gain  Gain=(Rsh+Rs)/Rsh
  Subsystem : Subsystem
  Subsystem1 : Subsystem
  U : Outport
  Isc : Outport  Port=2
  wires:
  Subsystem/2(Ipv) -> Add1/1
  G/1 -> Subsystem/1(G)
  T/1 -> Subsystem/2(T), Subsystem1/1(T)
  Subsystem1/1(Id) -> Add1/2
  I/1 -> Subsystem1/3(I), Gain3/1
  Gain3/1 -> Add1/3
  Add1/1 -> Gain1/1
  Gain1/1 -> Subsystem1/2(U), U/1
  Subsystem/1(Isc) -> Isc/1

== system Series_connected_PV_modules/PV module #8/Bypass diode ==
  I : Inport
  Bypass diode junction temperature : Constant  Value=298
  Bypass diode saturation current : Constant  Value=3.2e-6
  Divide4 : Product  Inputs=/*
  Gain1 : Gain  Gain=Rs_bypass
  Gain2 : Gain  Gain=-1
  Gain9 : Gain  Gain=1.5
  Math Function2 : Math  Operator=log  SaturateOnIntegerOverflow=on
  Product2 : Product  RndMeth=Zero
  Saturation1 : Saturate  UpperLimit=1e24  LowerLimit=0
  Subtract : Sum
  Subtract5 : Sum
  Thermal voltage : Subsystem
  Ubypass : Outport
  wires:
  Gain2/1 -> Ubypass/1
  Subtract/1 -> Gain2/1
  Saturation1/1 -> Gain1/1, Subtract5/2
  Subtract5/1 -> Divide4/2
  Divide4/1 -> Math Function2/1
  Bypass diode junction temperature/1 -> Thermal voltage/1(T)
  Gain1/1 -> Subtract/2
  Product2/1 -> Subtract/1
  I/1 -> Saturation1/1
  Bypass diode saturation current/1 -> Divide4/1, Subtract5/1
  Thermal voltage/1(Vt) -> Gain9/1
  Gain9/1 -> Product2/1
  Math Function2/1 -> Product2/2

== system Series_connected_PV_modules/PV module #8/Pv module ==
  G : Inport
  T : Inport  Port=2
  I : Inport  Port=3
  Add1 : Sum  Inputs=+--
  Gain1 : Gain  Gain=Rsh
  Gain3 : Gain  Gain=(Rsh+Rs)/Rsh
  Subsystem : Subsystem
  Subsystem1 : Subsystem
  U : Outport
  Isc : Outport  Port=2
  wires:
  Subsystem/1(Isc) -> Isc/1
  Gain1/1 -> U/1, Subsystem1/2(U)
  Add1/1 -> Gain1/1
  Gain3/1 -> Add1/3
  I/1 -> Gain3/1, Subsystem1/3(I)
  Subsystem1/1(Id) -> Add1/2
  T/1 -> Subsystem1/1(T), Subsystem/2(T)
  G/1 -> Subsystem/1(G)
  Subsystem/2(Ipv) -> Add1/1

== system Series_connected_PV_modules/PV module #9/Bypass diode ==
  I : Inport
  Bypass diode junction temperature : Constant  Value=298
  Bypass diode saturation current : Constant  Value=3.2e-6
  Divide4 : Product  Inputs=/*
  Gain1 : Gain  Gain=Rs_bypass
  Gain2 : Gain  Gain=-1
  Gain9 : Gain  Gain=1.5
  Math Function2 : Math  Operator=log  SaturateOnIntegerOverflow=on
  Product2 : Product  RndMeth=Zero
  Saturation1 : Saturate  UpperLimit=1e24  LowerLimit=0
  Subtract : Sum
  Subtract5 : Sum
  Thermal voltage : Subsystem
  Ubypass : Outport
  wires:
  Math Function2/1 -> Product2/2
  Gain9/1 -> Product2/1
  Thermal voltage/1(Vt) -> Gain9/1
  Bypass diode saturation current/1 -> Subtract5/1, Divide4/1
  I/1 -> Saturation1/1
  Product2/1 -> Subtract/1
  Gain1/1 -> Subtract/2
  Bypass diode junction temperature/1 -> Thermal voltage/1(T)
  Divide4/1 -> Math Function2/1
  Subtract5/1 -> Divide4/2
  Saturation1/1 -> Subtract5/2, Gain1/1
  Subtract/1 -> Gain2/1
  Gain2/1 -> Ubypass/1

== system Series_connected_PV_modules/PV module #9/Pv module ==
  G : Inport
  T : Inport  Port=2
  I : Inport  Port=3
  Add1 : Sum  Inputs=+--
  Gain1 : Gain  Gain=Rsh
  Gain3 : Gain  Gain=(Rsh+Rs)/Rsh
  Subsystem : Subsystem
  Subsystem1 : Subsystem
  U : Outport
  Isc : Outport  Port=2
  wires:
  Subsystem/2(Ipv) -> Add1/1
  G/1 -> Subsystem/1(G)
  T/1 -> Subsystem/2(T), Subsystem1/1(T)
  Subsystem1/1(Id) -> Add1/2
  I/1 -> Subsystem1/3(I), Gain3/1
  Gain3/1 -> Add1/3
  Add1/1 -> Gain1/1
  Gain1/1 -> Subsystem1/2(U), U/1
  Subsystem/1(Isc) -> Isc/1

== system Series_connected_PV_modules/PV module #1/Bypass diode/Thermal voltage ==
  T : Inport
  Constant5 : Constant  Value=k/q
  Product : Product  RndMeth=Zero
  Vt : Outport
  wires:
  Product/1 -> Vt/1
  T/1 -> Product/1
  Constant5/1 -> Product/2

== system Series_connected_PV_modules/PV module #1/Pv module/Subsystem ==
  G : Inport
  T : Inport  Port=2
  Add : Sum
  Constant : Constant  Value=Isc_stc
  Constant1 : Constant  Value=T_stc
  Constant2 : Constant  Value=G_stc
  Divide : Product  Inputs=*/
  Gain : Gain  Gain=Ki
  Gain1 : Gain  Gain=(Rsh+Rs)/Rsh
  Product1 : Product  RndMeth=Zero
  Subtract : Sum  Inputs=+-
  Isc : Outport
  Ipv : Outport  Port=2
  wires:
  Gain1/1 -> Ipv/1
  Product1/1 -> Isc/1, Gain1/1
  Divide/1 -> Product1/2
  Add/1 -> Product1/1
  G/1 -> Divide/1
  T/1 -> Subtract/1
  Constant2/1 -> Divide/2
  Subtract/1 -> Gain/1
  Constant1/1 -> Subtract/2
  Gain/1 -> Add/2
  Constant/1 -> Add/1

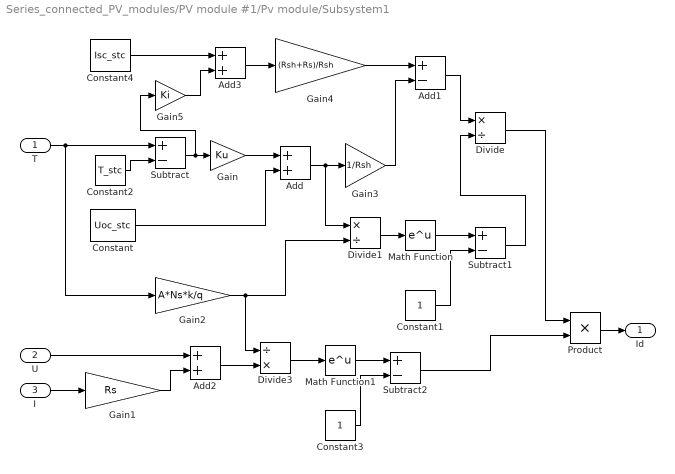
== system Series_connected_PV_modules/PV module #1/Pv module/Subsystem1 ==
  T : Inport
  U : Inport  Port=2
  I : Inport  Port=3
  Add : Sum
  Add1 : Sum  Inputs=+-
  Add2 : Sum
  Add3 : Sum
  Constant : Constant  Value=Uoc_stc
  Constant1 : Constant
  Constant2 : Constant  Value=T_stc
  Constant3 : Constant
  Constant4 : Constant  Value=Isc_stc
  Divide : Product  Inputs=*/
  Divide1 : Product  Inputs=*/
  Divide3 : Product  Inputs=/*
  Gain : Gain  Gain=Ku
  Gain1 : Gain  Gain=Rs
  Gain2 : Gain  Gain=A*Ns*k/q
  Gain3 : Gain  Gain=1/Rsh
  Gain4 : Gain  Gain=(Rsh+Rs)/Rsh
  Gain5 : Gain  Gain=Ki
  Math Function : Math  SaturateOnIntegerOverflow=on
  Math Function1 : Math  SaturateOnIntegerOverflow=on
  Product : Product  RndMeth=Zero
  Subtract : Sum  Inputs=+-
  Subtract1 : Sum  Inputs=+-
  Subtract2 : Sum  Inputs=+-
  Id : Outport
  wires:
  Gain4/1 -> Add1/1
  Subtract/1 -> Gain5/1, Gain/1
  Constant/1 -> Add/2
  Gain/1 -> Add/1
  Add3/1 -> Gain4/1
  Gain5/1 -> Add3/2
  Gain3/1 -> Add1/2
  Gain1/1 -> Add2/2
  I/1 -> Gain1/1
  Add/1 -> Gain3/1, Divide1/1
  Product/1 -> Id/1
  Subtract2/1 -> Product/2
  Constant3/1 -> Subtract2/2
  Math Function1/1 -> Subtract2/1
  Divide3/1 -> Math Function1/1
  Add2/1 -> Divide3/2
  U/1 -> Add2/1
  Divide/1 -> Product/1
  Subtract1/1 -> Divide/2
  Math Function/1 -> Subtract1/1
  Divide1/1 -> Math Function/1
  Gain2/1 -> Divide3/1, Divide1/2
  Constant1/1 -> Subtract1/2
  Add1/1 -> Divide/1
  T/1 -> Gain2/1, Subtract/1
  Constant2/1 -> Subtract/2
  Constant4/1 -> Add3/1

== system Series_connected_PV_modules/PV module #10/Bypass diode/Thermal voltage ==
  T : Inport
  Constant5 : Constant  Value=k/q
  Product : Product  RndMeth=Zero
  Vt : Outport
  wires:
  Product/1 -> Vt/1
  T/1 -> Product/1
  Constant5/1 -> Product/2

== system Series_connected_PV_modules/PV module #10/Pv module/Subsystem ==
  G : Inport
  T : Inport  Port=2
  Add : Sum
  Constant : Constant  Value=Isc_stc
  Constant1 : Constant  Value=T_stc
  Constant2 : Constant  Value=G_stc
  Divide : Product  Inputs=*/
  Gain : Gain  Gain=Ki
  Gain1 : Gain  Gain=(Rsh+Rs)/Rsh
  Product1 : Product  RndMeth=Zero
  Subtract : Sum  Inputs=+-
  Isc : Outport
  Ipv : Outport  Port=2
  wires:
  Gain1/1 -> Ipv/1
  Product1/1 -> Isc/1, Gain1/1
  Divide/1 -> Product1/2
  Add/1 -> Product1/1
  G/1 -> Divide/1
  T/1 -> Subtract/1
  Constant2/1 -> Divide/2
  Subtract/1 -> Gain/1
  Constant1/1 -> Subtract/2
  Gain/1 -> Add/2
  Constant/1 -> Add/1

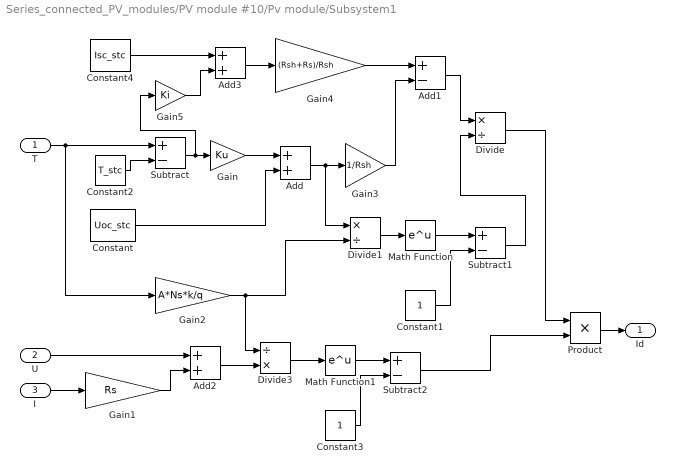
== system Series_connected_PV_modules/PV module #10/Pv module/Subsystem1 ==
  T : Inport
  U : Inport  Port=2
  I : Inport  Port=3
  Add : Sum
  Add1 : Sum  Inputs=+-
  Add2 : Sum
  Add3 : Sum
  Constant : Constant  Value=Uoc_stc
  Constant1 : Constant
  Constant2 : Constant  Value=T_stc
  Constant3 : Constant
  Constant4 : Constant  Value=Isc_stc
  Divide : Product  Inputs=*/
  Divide1 : Product  Inputs=*/
  Divide3 : Product  Inputs=/*
  Gain : Gain  Gain=Ku
  Gain1 : Gain  Gain=Rs
  Gain2 : Gain  Gain=A*Ns*k/q
  Gain3 : Gain  Gain=1/Rsh
  Gain4 : Gain  Gain=(Rsh+Rs)/Rsh
  Gain5 : Gain  Gain=Ki
  Math Function : Math  SaturateOnIntegerOverflow=on
  Math Function1 : Math  SaturateOnIntegerOverflow=on
  Product : Product  RndMeth=Zero
  Subtract : Sum  Inputs=+-
  Subtract1 : Sum  Inputs=+-
  Subtract2 : Sum  Inputs=+-
  Id : Outport
  wires:
  Gain4/1 -> Add1/1
  Subtract/1 -> Gain5/1, Gain/1
  Constant/1 -> Add/2
  Gain/1 -> Add/1
  Add3/1 -> Gain4/1
  Gain5/1 -> Add3/2
  Gain3/1 -> Add1/2
  Gain1/1 -> Add2/2
  I/1 -> Gain1/1
  Add/1 -> Gain3/1, Divide1/1
  Product/1 -> Id/1
  Subtract2/1 -> Product/2
  Constant3/1 -> Subtract2/2
  Math Function1/1 -> Subtract2/1
  Divide3/1 -> Math Function1/1
  Add2/1 -> Divide3/2
  U/1 -> Add2/1
  Divide/1 -> Product/1
  Subtract1/1 -> Divide/2
  Math Function/1 -> Subtract1/1
  Divide1/1 -> Math Function/1
  Gain2/1 -> Divide3/1, Divide1/2
  Constant1/1 -> Subtract1/2
  Add1/1 -> Divide/1
  T/1 -> Gain2/1, Subtract/1
  Constant2/1 -> Subtract/2
  Constant4/1 -> Add3/1

== system Series_connected_PV_modules/PV module #2/Bypass diode/Thermal voltage ==
  T : Inport
  Constant5 : Constant  Value=k/q
  Product : Product  RndMeth=Zero
  Vt : Outport
  wires:
  Constant5/1 -> Product/2
  T/1 -> Product/1
  Product/1 -> Vt/1

== system Series_connected_PV_modules/PV module #2/Pv module/Subsystem ==
  G : Inport
  T : Inport  Port=2
  Add : Sum
  Constant : Constant  Value=Isc_stc
  Constant1 : Constant  Value=T_stc
  Constant2 : Constant  Value=G_stc
  Divide : Product  Inputs=*/
  Gain : Gain  Gain=Ki
  Gain1 : Gain  Gain=(Rsh+Rs)/Rsh
  Product1 : Product  RndMeth=Zero
  Subtract : Sum  Inputs=+-
  Isc : Outport
  Ipv : Outport  Port=2
  wires:
  Constant/1 -> Add/1
  Gain/1 -> Add/2
  Constant1/1 -> Subtract/2
  Subtract/1 -> Gain/1
  Constant2/1 -> Divide/2
  T/1 -> Subtract/1
  G/1 -> Divide/1
  Add/1 -> Product1/1
  Divide/1 -> Product1/2
  Product1/1 -> Gain1/1, Isc/1
  Gain1/1 -> Ipv/1

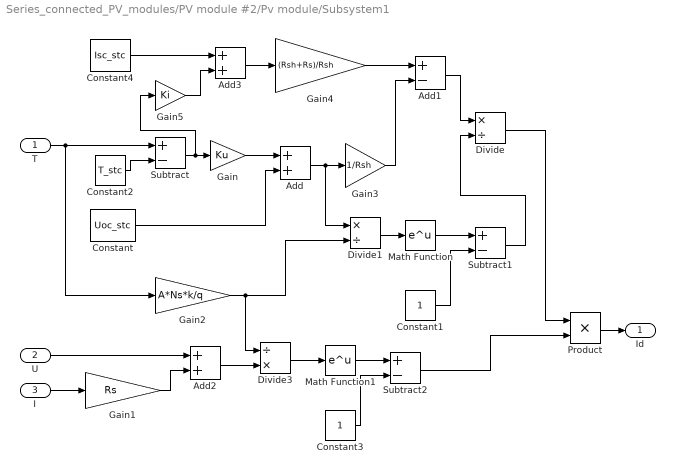
== system Series_connected_PV_modules/PV module #2/Pv module/Subsystem1 ==
  T : Inport
  U : Inport  Port=2
  I : Inport  Port=3
  Add : Sum
  Add1 : Sum  Inputs=+-
  Add2 : Sum
  Add3 : Sum
  Constant : Constant  Value=Uoc_stc
  Constant1 : Constant
  Constant2 : Constant  Value=T_stc
  Constant3 : Constant
  Constant4 : Constant  Value=Isc_stc
  Divide : Product  Inputs=*/
  Divide1 : Product  Inputs=*/
  Divide3 : Product  Inputs=/*
  Gain : Gain  Gain=Ku
  Gain1 : Gain  Gain=Rs
  Gain2 : Gain  Gain=A*Ns*k/q
  Gain3 : Gain  Gain=1/Rsh
  Gain4 : Gain  Gain=(Rsh+Rs)/Rsh
  Gain5 : Gain  Gain=Ki
  Math Function : Math  SaturateOnIntegerOverflow=on
  Math Function1 : Math  SaturateOnIntegerOverflow=on
  Product : Product  RndMeth=Zero
  Subtract : Sum  Inputs=+-
  Subtract1 : Sum  Inputs=+-
  Subtract2 : Sum  Inputs=+-
  Id : Outport
  wires:
  Constant4/1 -> Add3/1
  Constant2/1 -> Subtract/2
  T/1 -> Subtract/1, Gain2/1
  Add1/1 -> Divide/1
  Constant1/1 -> Subtract1/2
  Gain2/1 -> Divide1/2, Divide3/1
  Divide1/1 -> Math Function/1
  Math Function/1 -> Subtract1/1
  Subtract1/1 -> Divide/2
  Divide/1 -> Product/1
  U/1 -> Add2/1
  Add2/1 -> Divide3/2
  Divide3/1 -> Math Function1/1
  Math Function1/1 -> Subtract2/1
  Constant3/1 -> Subtract2/2
  Subtract2/1 -> Product/2
  Product/1 -> Id/1
  Add/1 -> Divide1/1, Gain3/1
  I/1 -> Gain1/1
  Gain1/1 -> Add2/2
  Gain3/1 -> Add1/2
  Gain5/1 -> Add3/2
  Add3/1 -> Gain4/1
  Gain/1 -> Add/1
  Constant/1 -> Add/2
  Subtract/1 -> Gain/1, Gain5/1
  Gain4/1 -> Add1/1

== system Series_connected_PV_modules/PV module #3/Bypass diode/Thermal voltage ==
  T : Inport
  Constant5 : Constant  Value=k/q
  Product : Product  RndMeth=Zero
  Vt : Outport
  wires:
  Product/1 -> Vt/1
  T/1 -> Product/1
  Constant5/1 -> Product/2

== system Series_connected_PV_modules/PV module #3/Pv module/Subsystem ==
  G : Inport
  T : Inport  Port=2
  Add : Sum
  Constant : Constant  Value=Isc_stc
  Constant1 : Constant  Value=T_stc
  Constant2 : Constant  Value=G_stc
  Divide : Product  Inputs=*/
  Gain : Gain  Gain=Ki
  Gain1 : Gain  Gain=(Rsh+Rs)/Rsh
  Product1 : Product  RndMeth=Zero
  Subtract : Sum  Inputs=+-
  Isc : Outport
  Ipv : Outport  Port=2
  wires:
  Gain1/1 -> Ipv/1
  Product1/1 -> Isc/1, Gain1/1
  Divide/1 -> Product1/2
  Add/1 -> Product1/1
  G/1 -> Divide/1
  T/1 -> Subtract/1
  Constant2/1 -> Divide/2
  Subtract/1 -> Gain/1
  Constant1/1 -> Subtract/2
  Gain/1 -> Add/2
  Constant/1 -> Add/1

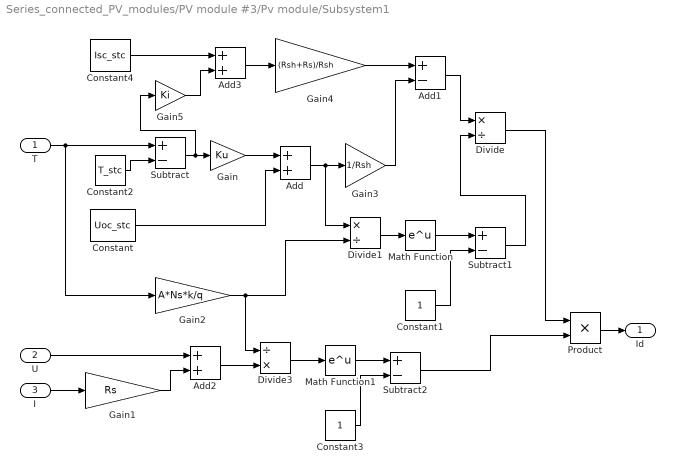
== system Series_connected_PV_modules/PV module #3/Pv module/Subsystem1 ==
  T : Inport
  U : Inport  Port=2
  I : Inport  Port=3
  Add : Sum
  Add1 : Sum  Inputs=+-
  Add2 : Sum
  Add3 : Sum
  Constant : Constant  Value=Uoc_stc
  Constant1 : Constant
  Constant2 : Constant  Value=T_stc
  Constant3 : Constant
  Constant4 : Constant  Value=Isc_stc
  Divide : Product  Inputs=*/
  Divide1 : Product  Inputs=*/
  Divide3 : Product  Inputs=/*
  Gain : Gain  Gain=Ku
  Gain1 : Gain  Gain=Rs
  Gain2 : Gain  Gain=A*Ns*k/q
  Gain3 : Gain  Gain=1/Rsh
  Gain4 : Gain  Gain=(Rsh+Rs)/Rsh
  Gain5 : Gain  Gain=Ki
  Math Function : Math  SaturateOnIntegerOverflow=on
  Math Function1 : Math  SaturateOnIntegerOverflow=on
  Product : Product  RndMeth=Zero
  Subtract : Sum  Inputs=+-
  Subtract1 : Sum  Inputs=+-
  Subtract2 : Sum  Inputs=+-
  Id : Outport
  wires:
  Gain4/1 -> Add1/1
  Subtract/1 -> Gain5/1, Gain/1
  Constant/1 -> Add/2
  Gain/1 -> Add/1
  Add3/1 -> Gain4/1
  Gain5/1 -> Add3/2
  Gain3/1 -> Add1/2
  Gain1/1 -> Add2/2
  I/1 -> Gain1/1
  Add/1 -> Gain3/1, Divide1/1
  Product/1 -> Id/1
  Subtract2/1 -> Product/2
  Constant3/1 -> Subtract2/2
  Math Function1/1 -> Subtract2/1
  Divide3/1 -> Math Function1/1
  Add2/1 -> Divide3/2
  U/1 -> Add2/1
  Divide/1 -> Product/1
  Subtract1/1 -> Divide/2
  Math Function/1 -> Subtract1/1
  Divide1/1 -> Math Function/1
  Gain2/1 -> Divide3/1, Divide1/2
  Constant1/1 -> Subtract1/2
  Add1/1 -> Divide/1
  T/1 -> Gain2/1, Subtract/1
  Constant2/1 -> Subtract/2
  Constant4/1 -> Add3/1

== system Series_connected_PV_modules/PV module #4/Bypass diode/Thermal voltage ==
  T : Inport
  Constant5 : Constant  Value=k/q
  Product : Product  RndMeth=Zero
  Vt : Outport
  wires:
  Constant5/1 -> Product/2
  T/1 -> Product/1
  Product/1 -> Vt/1

== system Series_connected_PV_modules/PV module #4/Pv module/Subsystem ==
  G : Inport
  T : Inport  Port=2
  Add : Sum
  Constant : Constant  Value=Isc_stc
  Constant1 : Constant  Value=T_stc
  Constant2 : Constant  Value=G_stc
  Divide : Product  Inputs=*/
  Gain : Gain  Gain=Ki
  Gain1 : Gain  Gain=(Rsh+Rs)/Rsh
  Product1 : Product  RndMeth=Zero
  Subtract : Sum  Inputs=+-
  Isc : Outport
  Ipv : Outport  Port=2
  wires:
  Constant/1 -> Add/1
  Gain/1 -> Add/2
  Constant1/1 -> Subtract/2
  Subtract/1 -> Gain/1
  Constant2/1 -> Divide/2
  T/1 -> Subtract/1
  G/1 -> Divide/1
  Add/1 -> Product1/1
  Divide/1 -> Product1/2
  Product1/1 -> Gain1/1, Isc/1
  Gain1/1 -> Ipv/1

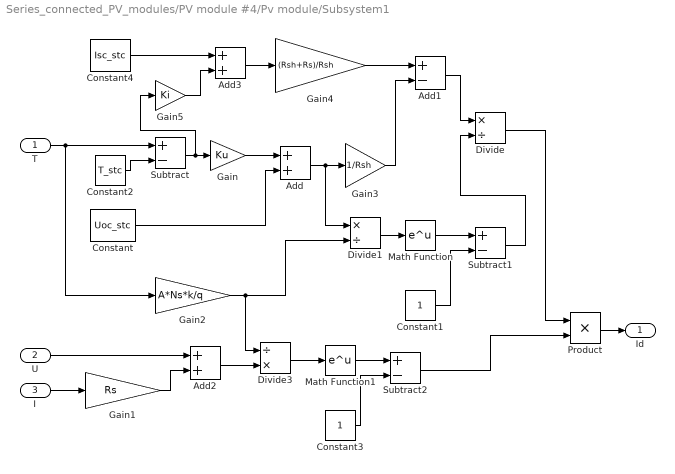
== system Series_connected_PV_modules/PV module #4/Pv module/Subsystem1 ==
  T : Inport
  U : Inport  Port=2
  I : Inport  Port=3
  Add : Sum
  Add1 : Sum  Inputs=+-
  Add2 : Sum
  Add3 : Sum
  Constant : Constant  Value=Uoc_stc
  Constant1 : Constant
  Constant2 : Constant  Value=T_stc
  Constant3 : Constant
  Constant4 : Constant  Value=Isc_stc
  Divide : Product  Inputs=*/
  Divide1 : Product  Inputs=*/
  Divide3 : Product  Inputs=/*
  Gain : Gain  Gain=Ku
  Gain1 : Gain  Gain=Rs
  Gain2 : Gain  Gain=A*Ns*k/q
  Gain3 : Gain  Gain=1/Rsh
  Gain4 : Gain  Gain=(Rsh+Rs)/Rsh
  Gain5 : Gain  Gain=Ki
  Math Function : Math  SaturateOnIntegerOverflow=on
  Math Function1 : Math  SaturateOnIntegerOverflow=on
  Product : Product  RndMeth=Zero
  Subtract : Sum  Inputs=+-
  Subtract1 : Sum  Inputs=+-
  Subtract2 : Sum  Inputs=+-
  Id : Outport
  wires:
  Constant4/1 -> Add3/1
  Constant2/1 -> Subtract/2
  T/1 -> Subtract/1, Gain2/1
  Add1/1 -> Divide/1
  Constant1/1 -> Subtract1/2
  Gain2/1 -> Divide1/2, Divide3/1
  Divide1/1 -> Math Function/1
  Math Function/1 -> Subtract1/1
  Subtract1/1 -> Divide/2
  Divide/1 -> Product/1
  U/1 -> Add2/1
  Add2/1 -> Divide3/2
  Divide3/1 -> Math Function1/1
  Math Function1/1 -> Subtract2/1
  Constant3/1 -> Subtract2/2
  Subtract2/1 -> Product/2
  Product/1 -> Id/1
  Add/1 -> Divide1/1, Gain3/1
  I/1 -> Gain1/1
  Gain1/1 -> Add2/2
  Gain3/1 -> Add1/2
  Gain5/1 -> Add3/2
  Add3/1 -> Gain4/1
  Gain/1 -> Add/1
  Constant/1 -> Add/2
  Subtract/1 -> Gain/1, Gain5/1
  Gain4/1 -> Add1/1

== system Series_connected_PV_modules/PV module #5/Bypass diode/Thermal voltage ==
  T : Inport
  Constant5 : Constant  Value=k/q
  Product : Product  RndMeth=Zero
  Vt : Outport
  wires:
  Product/1 -> Vt/1
  T/1 -> Product/1
  Constant5/1 -> Product/2

== system Series_connected_PV_modules/PV module #5/Pv module/Subsystem ==
  G : Inport
  T : Inport  Port=2
  Add : Sum
  Constant : Constant  Value=Isc_stc
  Constant1 : Constant  Value=T_stc
  Constant2 : Constant  Value=G_stc
  Divide : Product  Inputs=*/
  Gain : Gain  Gain=Ki
  Gain1 : Gain  Gain=(Rsh+Rs)/Rsh
  Product1 : Product  RndMeth=Zero
  Subtract : Sum  Inputs=+-
  Isc : Outport
  Ipv : Outport  Port=2
  wires:
  Gain1/1 -> Ipv/1
  Product1/1 -> Isc/1, Gain1/1
  Divide/1 -> Product1/2
  Add/1 -> Product1/1
  G/1 -> Divide/1
  T/1 -> Subtract/1
  Constant2/1 -> Divide/2
  Subtract/1 -> Gain/1
  Constant1/1 -> Subtract/2
  Gain/1 -> Add/2
  Constant/1 -> Add/1

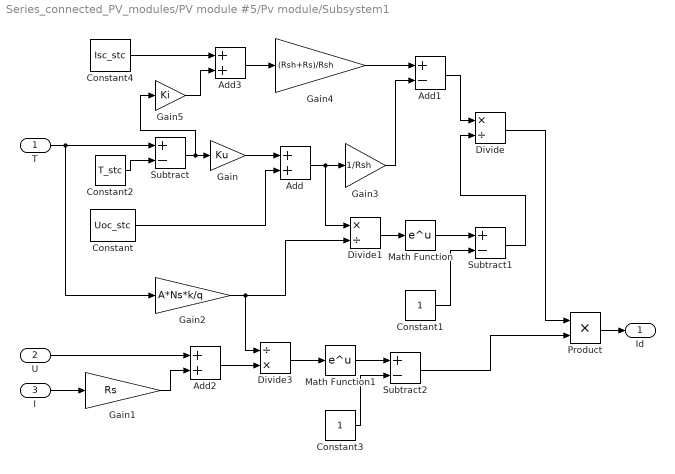
== system Series_connected_PV_modules/PV module #5/Pv module/Subsystem1 ==
  T : Inport
  U : Inport  Port=2
  I : Inport  Port=3
  Add : Sum
  Add1 : Sum  Inputs=+-
  Add2 : Sum
  Add3 : Sum
  Constant : Constant  Value=Uoc_stc
  Constant1 : Constant
  Constant2 : Constant  Value=T_stc
  Constant3 : Constant
  Constant4 : Constant  Value=Isc_stc
  Divide : Product  Inputs=*/
  Divide1 : Product  Inputs=*/
  Divide3 : Product  Inputs=/*
  Gain : Gain  Gain=Ku
  Gain1 : Gain  Gain=Rs
  Gain2 : Gain  Gain=A*Ns*k/q
  Gain3 : Gain  Gain=1/Rsh
  Gain4 : Gain  Gain=(Rsh+Rs)/Rsh
  Gain5 : Gain  Gain=Ki
  Math Function : Math  SaturateOnIntegerOverflow=on
  Math Function1 : Math  SaturateOnIntegerOverflow=on
  Product : Product  RndMeth=Zero
  Subtract : Sum  Inputs=+-
  Subtract1 : Sum  Inputs=+-
  Subtract2 : Sum  Inputs=+-
  Id : Outport
  wires:
  Gain4/1 -> Add1/1
  Subtract/1 -> Gain5/1, Gain/1
  Constant/1 -> Add/2
  Gain/1 -> Add/1
  Add3/1 -> Gain4/1
  Gain5/1 -> Add3/2
  Gain3/1 -> Add1/2
  Gain1/1 -> Add2/2
  I/1 -> Gain1/1
  Add/1 -> Gain3/1, Divide1/1
  Product/1 -> Id/1
  Subtract2/1 -> Product/2
  Constant3/1 -> Subtract2/2
  Math Function1/1 -> Subtract2/1
  Divide3/1 -> Math Function1/1
  Add2/1 -> Divide3/2
  U/1 -> Add2/1
  Divide/1 -> Product/1
  Subtract1/1 -> Divide/2
  Math Function/1 -> Subtract1/1
  Divide1/1 -> Math Function/1
  Gain2/1 -> Divide3/1, Divide1/2
  Constant1/1 -> Subtract1/2
  Add1/1 -> Divide/1
  T/1 -> Gain2/1, Subtract/1
  Constant2/1 -> Subtract/2
  Constant4/1 -> Add3/1

== system Series_connected_PV_modules/PV module #6/Bypass diode/Thermal voltage ==
  T : Inport
  Constant5 : Constant  Value=k/q
  Product : Product  RndMeth=Zero
  Vt : Outport
  wires:
  Constant5/1 -> Product/2
  T/1 -> Product/1
  Product/1 -> Vt/1

== system Series_connected_PV_modules/PV module #6/Pv module/Subsystem ==
  G : Inport
  T : Inport  Port=2
  Add : Sum
  Constant : Constant  Value=Isc_stc
  Constant1 : Constant  Value=T_stc
  Constant2 : Constant  Value=G_stc
  Divide : Product  Inputs=*/
  Gain : Gain  Gain=Ki
  Gain1 : Gain  Gain=(Rsh+Rs)/Rsh
  Product1 : Product  RndMeth=Zero
  Subtract : Sum  Inputs=+-
  Isc : Outport
  Ipv : Outport  Port=2
  wires:
  Constant/1 -> Add/1
  Gain/1 -> Add/2
  Constant1/1 -> Subtract/2
  Subtract/1 -> Gain/1
  Constant2/1 -> Divide/2
  T/1 -> Subtract/1
  G/1 -> Divide/1
  Add/1 -> Product1/1
  Divide/1 -> Product1/2
  Product1/1 -> Gain1/1, Isc/1
  Gain1/1 -> Ipv/1

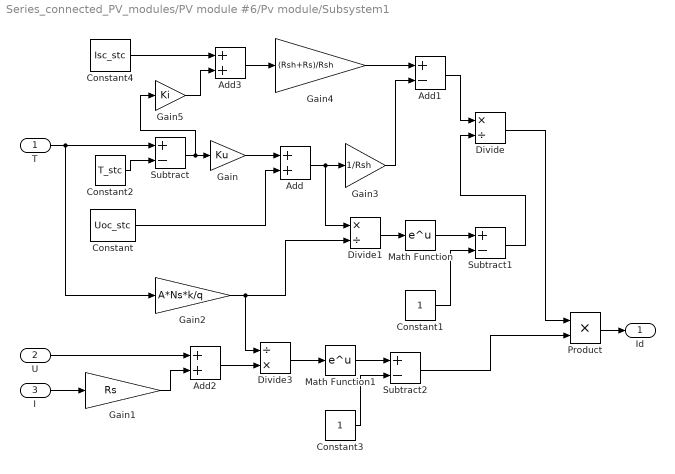
== system Series_connected_PV_modules/PV module #6/Pv module/Subsystem1 ==
  T : Inport
  U : Inport  Port=2
  I : Inport  Port=3
  Add : Sum
  Add1 : Sum  Inputs=+-
  Add2 : Sum
  Add3 : Sum
  Constant : Constant  Value=Uoc_stc
  Constant1 : Constant
  Constant2 : Constant  Value=T_stc
  Constant3 : Constant
  Constant4 : Constant  Value=Isc_stc
  Divide : Product  Inputs=*/
  Divide1 : Product  Inputs=*/
  Divide3 : Product  Inputs=/*
  Gain : Gain  Gain=Ku
  Gain1 : Gain  Gain=Rs
  Gain2 : Gain  Gain=A*Ns*k/q
  Gain3 : Gain  Gain=1/Rsh
  Gain4 : Gain  Gain=(Rsh+Rs)/Rsh
  Gain5 : Gain  Gain=Ki
  Math Function : Math  SaturateOnIntegerOverflow=on
  Math Function1 : Math  SaturateOnIntegerOverflow=on
  Product : Product  RndMeth=Zero
  Subtract : Sum  Inputs=+-
  Subtract1 : Sum  Inputs=+-
  Subtract2 : Sum  Inputs=+-
  Id : Outport
  wires:
  Constant4/1 -> Add3/1
  Constant2/1 -> Subtract/2
  T/1 -> Subtract/1, Gain2/1
  Add1/1 -> Divide/1
  Constant1/1 -> Subtract1/2
  Gain2/1 -> Divide1/2, Divide3/1
  Divide1/1 -> Math Function/1
  Math Function/1 -> Subtract1/1
  Subtract1/1 -> Divide/2
  Divide/1 -> Product/1
  U/1 -> Add2/1
  Add2/1 -> Divide3/2
  Divide3/1 -> Math Function1/1
  Math Function1/1 -> Subtract2/1
  Constant3/1 -> Subtract2/2
  Subtract2/1 -> Product/2
  Product/1 -> Id/1
  Add/1 -> Divide1/1, Gain3/1
  I/1 -> Gain1/1
  Gain1/1 -> Add2/2
  Gain3/1 -> Add1/2
  Gain5/1 -> Add3/2
  Add3/1 -> Gain4/1
  Gain/1 -> Add/1
  Constant/1 -> Add/2
  Subtract/1 -> Gain/1, Gain5/1
  Gain4/1 -> Add1/1

== system Series_connected_PV_modules/PV module #7/Bypass diode/Thermal voltage ==
  T : Inport
  Constant5 : Constant  Value=k/q
  Product : Product  RndMeth=Zero
  Vt : Outport
  wires:
  Constant5/1 -> Product/2
  T/1 -> Product/1
  Product/1 -> Vt/1

== system Series_connected_PV_modules/PV module #7/Pv module/Subsystem ==
  G : Inport
  T : Inport  Port=2
  Add : Sum
  Constant : Constant  Value=Isc_stc
  Constant1 : Constant  Value=T_stc
  Constant2 : Constant  Value=G_stc
  Divide : Product  Inputs=*/
  Gain : Gain  Gain=Ki
  Gain1 : Gain  Gain=(Rsh+Rs)/Rsh
  Product1 : Product  RndMeth=Zero
  Subtract : Sum  Inputs=+-
  Isc : Outport
  Ipv : Outport  Port=2
  wires:
  Constant/1 -> Add/1
  Gain/1 -> Add/2
  Constant1/1 -> Subtract/2
  Subtract/1 -> Gain/1
  Constant2/1 -> Divide/2
  T/1 -> Subtract/1
  G/1 -> Divide/1
  Add/1 -> Product1/1
  Divide/1 -> Product1/2
  Product1/1 -> Gain1/1, Isc/1
  Gain1/1 -> Ipv/1
